simulink model "uavCtrl"  (R2018b)
settings: Solver=VariableStepAuto  StartTime=0.0  StopTime=10  RelTol=1e-3  EnableMultiTasking=on
settings Model: Creator=Administrator  LastModifiedBy=win-s
settings DataIOCC: LimitDataPoints=on  SaveFormat=Array  SignalLoggingSaveFormat=ModelDataLogs
settings OptimizationCC: ExpressionDepthLimit=2147483647  InitFltsAndDblsToZero=on  LifeSpan=inf
settings DebuggingCC: UnderspecifiedInitializationDetection=Classic  MergeDetectMultiDrivingBlocksExec=none  SolverPrmCheckMsg=warning  FcnCallInpInsideContextMsg=warning  StateNameClashWarn=warning  SFUnexpectedBacktrackingDiag=warning  SFNoUnconditionalDefaultTransitionDiag=warning
settings HardwareCC: ProdBitPerPointer=32  ProdBitPerSizeT=32  ProdBitPerPtrDiffT=32  ProdLargestAtomicFloat=None  ProdIntDivRoundTo=Undefined  ProdEndianess=Unspecified  ProdWordSize=32  ProdHWDeviceType=32-bit Generic
settings ModelReferenceCC: PropagateSignalLabelsOutOfModel=off
settings SFSimCC: SimUseLocalCustomCode=off
settings RTWCC: RTWUseLocalCustomCode=off
settings CodeAppCC: StateflowObjectComments=on
settings GRTTargetCC: TargetLangStandard=C89/C90 (ANSI)  CombineOutputUpdateFcns=off  GRTInterface=on
settings ConfigComp: CovMetricSettings=dw  CovHtmlReporting=on  CovSaveCumulativeToWorkspaceVar=on  CovSaveSingleToWorkspaceVar=on  CovExternalEMLEnable=off

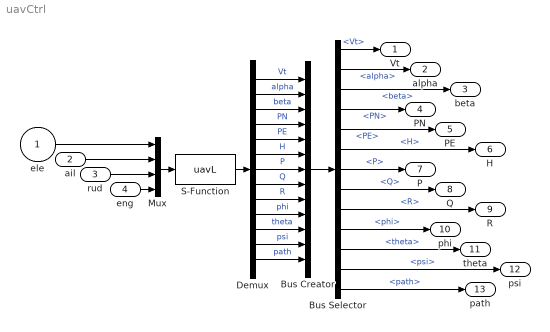
== system uavCtrl ==
  ele : Inport
  ail : Inport  Port=2
  rud : Inport  Port=3
  eng : Inport  Port=4
  Bus Creator : BusCreator  Inputs=13
  Bus Selector : BusSelector  OutputSignals=Vt,alpha,beta,PN,PE,H,P,Q,R,phi,theta,psi,path
  Demux : Demux  Outputs=13
  Mux : Mux
  S-Function : S-Function  FunctionName=uavL  SFunctionDeploymentMode=off  EnableBusSupport=off
  Vt : Outport
  alpha : Outport  Port=2
  beta : Outport  Port=3
  PN : Outport  Port=4
  PE : Outport  Port=5
  H : Outport  Port=6
  P : Outport  Port=7
  Q : Outport  Port=8
  R : Outport  Port=9
  phi : Outport  Port=10
  theta : Outport  Port=11
  psi : Outport  Port=12
  path : Outport  Port=13
  wires:
  S-Function/1 -> Demux/1
  Demux/1 -> Bus Creator/1  "Vt"
  Demux/2 -> Bus Creator/2  "alpha"
  Demux/3 -> Bus Creator/3  "beta"
  Demux/4 -> Bus Creator/4  "PN"
  Demux/5 -> Bus Creator/5  "PE"
  Demux/6 -> Bus Creator/6  "H"
  Demux/7 -> Bus Creator/7  "P"
  Demux/8 -> Bus Creator/8  "Q"
  Demux/9 -> Bus Creator/9  "R"
  Demux/10 -> Bus Creator/10  "phi"
  Demux/11 -> Bus Creator/11  "theta"
  Demux/12 -> Bus Creator/12  "psi"
  Demux/13 -> Bus Creator/13  "path"
  Bus Creator/1 -> Bus Selector/1
  Bus Selector/1 -> Vt/1  "<Vt>"
  Bus Selector/2 -> alpha/1  "<alpha>"
  Bus Selector/3 -> beta/1  "<beta>"
  Bus Selector/4 -> PN/1  "<PN>"
  Bus Selector/13 -> path/1  "<path>"
  Bus Selector/12 -> psi/1  "<psi>"
  Bus Selector/11 -> theta/1  "<theta>"
  Bus Selector/10 -> phi/1  "<phi>"
  Bus Selector/9 -> R/1  "<R>"
  Bus Selector/8 -> Q/1  "<Q>"
  Bus Selector/7 -> P/1  "<P>"
  Bus Selector/6 -> H/1  "<H>"
  Bus Selector/5 -> PE/1  "<PE>"
  Mux/1 -> S-Function/1
  ail/1 -> Mux/2
  ele/1 -> Mux/1
  rud/1 -> Mux/3
  eng/1 -> Mux/4
